simulink model "Bai30"  (R2020a)
settings: Solver=VariableStepAuto  StartTime=0.0  StopTime=10.0  RelTol=1e-3
settings Model: Creator=NgocNguyen  LastModifiedBy=NgocNguyen

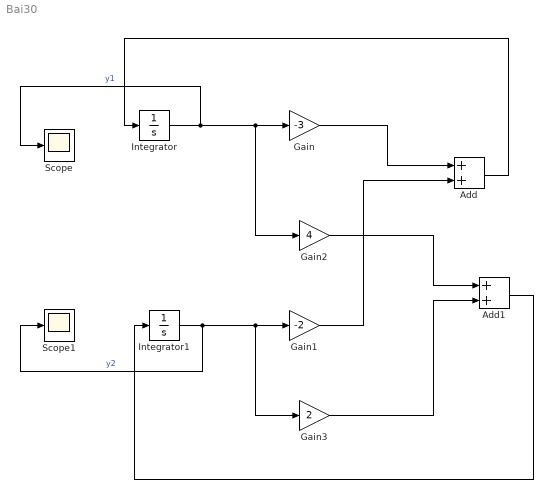
== system Bai30 ==
  Add : Sum
  Add1 : Sum
  Gain : Gain  Gain=-3
  Gain1 : Gain  Gain=-2
  Gain2 : Gain  Gain=4
  Gain3 : Gain  Gain=2
  Integrator : Integrator  InitialCondition=1
  Integrator1 : Integrator  InitialCondition=1
  Scope : Scope
  Scope1 : Scope
  wires:
  Integrator/1 -> Scope/1, Gain2/1, Gain/1  "y1"
  Gain/1 -> Add/1
  Integrator1/1 -> Scope1/1, Gain3/1, Gain1/1  "y2"
  Gain1/1 -> Add/2
  Gain2/1 -> Add1/1
  Gain3/1 -> Add1/2
  Add1/1 -> Integrator1/1
  Add/1 -> Integrator/1
